simulink model "assigment3_3_3"  (R2021b)
settings: Solver=FixedStepAuto  StartTime=0.0  StopTime=100  FixedStep=0.001  RelTol=1e-3
settings Model: Creator=fatima mn  LastModifiedBy=fatima mn

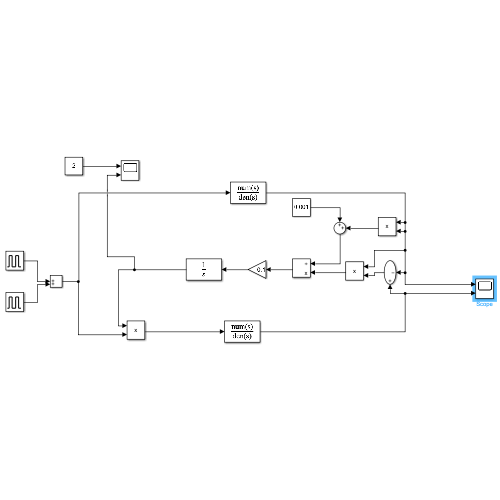
[thumbnail: Simulink's stored preview of the top-level diagram]
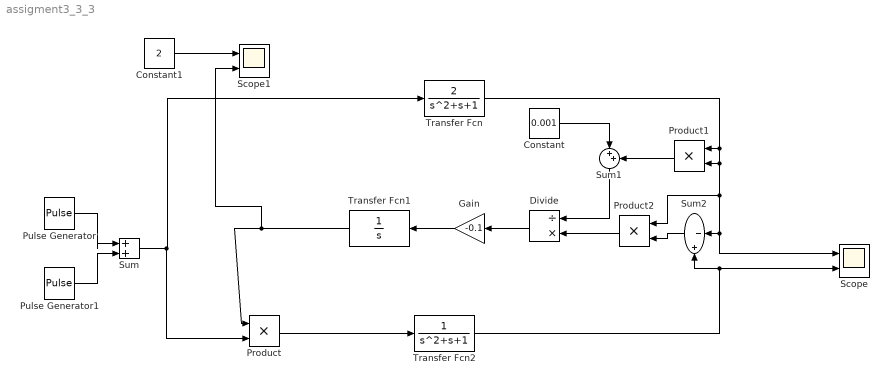
== system assigment3_3_3 ==
  Constant : Constant  Value=0.001
  Constant1 : Constant  Value=2
  Divide : Product  Inputs=/*
  Gain : Gain  Gain=-0.1
  Product : Product
  Product1 : Product
  Product2 : Product
  Pulse Generator : DiscretePulseGenerator  PulseType=Time based  Amplitude=3.5  Period=20  PulseWidth=50
  Pulse Generator1 : DiscretePulseGenerator  PulseType=Time based  Amplitude=-3.5  Period=20  PulseWidth=50  PhaseDelay=10
  Scope : Scope  NumInputPorts=2
  Scope1 : Scope  NumInputPorts=2
  Sum : Sum  Inputs=|++
  Sum1 : Sum  Inputs=|++
  Sum2 : Sum  Inputs=|-+
  Transfer Fcn : TransferFcn  Numerator=[2]  Denominator=[1 1 1]
  Transfer Fcn1 : TransferFcn  Denominator=[1 0]
  Transfer Fcn2 : TransferFcn  Denominator=[1 1 1]
  wires:
  Pulse Generator/1 -> Sum/1
  Pulse Generator1/1 -> Sum/2
  Sum/1 -> Product/2, Transfer Fcn/1
  Gain/1 -> Transfer Fcn1/1
  Divide/1 -> Gain/1
  Transfer Fcn1/1 -> Scope1/2, Product/1
  Product/1 -> Transfer Fcn2/1
  Product1/1 -> Sum1/2
  Constant/1 -> Sum1/1
  Sum1/1 -> Divide/1
  Product2/1 -> Divide/2
  Sum2/1 -> Product2/2
  Transfer Fcn2/1 -> Scope/2, Sum2/2
  Transfer Fcn/1 -> Product1/2, Product2/1, Scope/1, Sum2/1, Product1/1
  Constant1/1 -> Scope1/1
